simulink library "Code_Gen_lib"  (R2023a)
settings: Solver=VariableStepAuto  StartTime=0.0  StopTime=10.0  RelTol=1e-3
libraries: Autonomous_lib x1, Disabled_lib x1, Swerve_Drive_lib x1, Teleop_lib x1, Test_lib x1
settings Model: Creator=FIRSTMentor  LastModifiedBy=FIRSTMentor

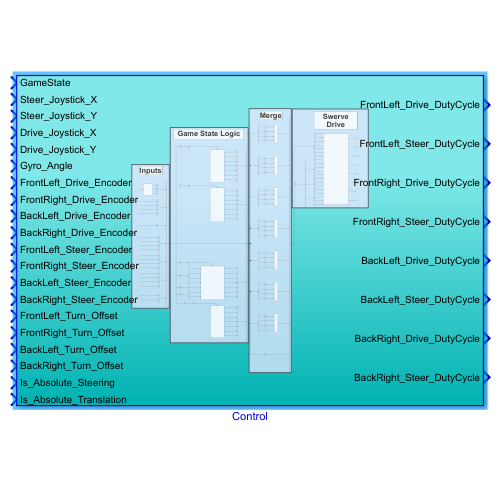
[thumbnail: Simulink's stored preview of the top-level diagram]
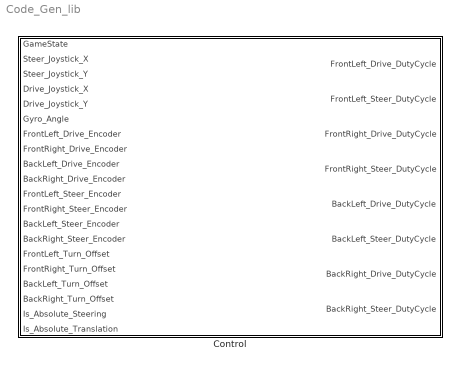
== system Code_Gen_lib ==
  Control : Subsystem

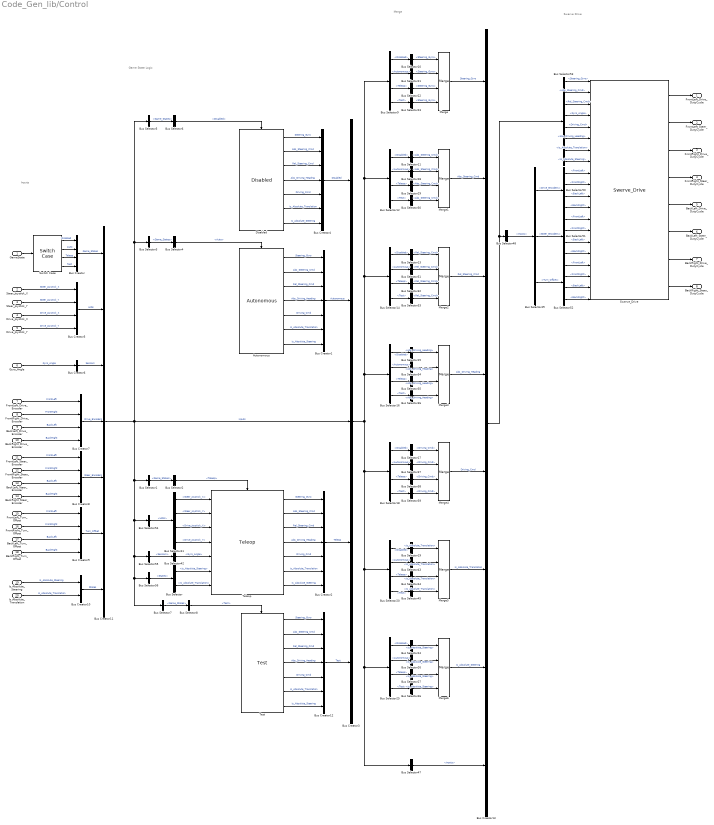
== system Code_Gen_lib/Control ==
  note: Game State Logic
  note: Merge
  note: Swerve Drive
  note: Inputs
  GameState : Inport
  Steer_Joystick_X : Inport  Port=2
  Steer_Joystick_Y : Inport  Port=3
  Drive_Joystick_X : Inport  Port=4
  Drive_Joystick_Y : Inport  Port=5
  Gyro_Angle : Inport  Port=6
  FrontLeft_Drive_Encoder : Inport  Port=7
  FrontRight_Drive_Encoder : Inport  Port=8
  BackLeft_Drive_Encoder : Inport  Port=9
  BackRight_Drive_Encoder : Inport  Port=10
  FrontLeft_Steer_Encoder : Inport  Port=11
  FrontRight_Steer_Encoder : Inport  Port=12
  BackLeft_Steer_Encoder : Inport  Port=13
  BackRight_Steer_Encoder : Inport  Port=14
  FrontLeft_Turn_Offset : Inport  Port=15
  FrontRight_Turn_Offset : Inport  Port=16
  BackLeft_Turn_Offset : Inport  Port=17
  BackRight_Turn_Offset : Inport  Port=18
  Is_Absolute_Steering : Inport  Port=19
  Is_Absolute_Translation : Inport  Port=20
  Autonomous : Autonomous_lib/Autonomous  SystemSampleTime=-1  VariantActivationTime=update diagram  Latency=0  AutoFrameSizeCalculation=off
  Bus Creator{,5,7..9} (5 alike) : BusCreator  Inputs=4
  Bus Creator{1..2,4,11..12} (5 alike) : BusCreator  Inputs=7
  Bus Creator10 : BusCreator  Inputs=2
  Bus Creator13 : BusCreator  Inputs=8
  Bus Creator3 : BusCreator  Inputs=5
  Bus Creator6 : BusCreator  Inputs=1
  Bus Selector : BusSelector  OutputSignals=Is_Absolute_Steering,Is_Absolute_Translation
  Bus Selector{1,3,5,7} (4 alike) : BusSelector  OutputSignals=Game_States
  Bus Selector{10,21..23} (4 alike) : BusSelector  OutputSignals=Steering_Gyro
  Bus Selector{11,28..30} (4 alike) : BusSelector  OutputSignals=Abs_Steering_Cmd
  Bus Selector{9,12,14,16,18,20,25} (7 alike) : BusSelector  OutputSignals=Disabled,Autonomous,Teleop,Test
  Bus Selector{13,31..33} (4 alike) : BusSelector  OutputSignals=Rel_Steering_Cmd
  Bus Selector{15,34..36} (4 alike) : BusSelector  OutputSignals=Abs_Driving_Heading
  Bus Selector{17,37..39} (4 alike) : BusSelector  OutputSignals=Driving_Cmd
  Bus Selector{19,43..45} (4 alike) : BusSelector  OutputSignals=Is_Absolute_Translation
  Bus Selector2 : BusSelector  OutputSignals=Teleop
  Bus Selector{24,26..27,46} (4 alike) : BusSelector  OutputSignals=Is_Absolute_Steering
  Bus Selector4 : BusSelector  OutputSignals=Auto
  Bus Selector41 : BusSelector  OutputSignals=Steer_Joystick_X,Steer_Joystick_Y,Drive_Joystick_X,Drive_Joystick_Y
  Bus Selector42 : BusSelector  OutputSignals=Gyro_Angle
  Bus Selector47 : BusSelector  OutputSignals=Inputs
  Bus Selector48 : BusSelector  OutputSignals=Inputs
  Bus Selector49 : BusSelector  OutputSignals=Drive_Encoders,Steer_Encoders,Turn_Offset
  Bus Selector50 : BusSelector  OutputSignals=FrontLeft,FrontRight,BackLeft,BackRight
  Bus Selector51 : BusSelector  OutputSignals=FrontLeft,FrontRight,BackLeft,BackRight
  Bus Selector52 : BusSelector  OutputSignals=FrontLeft,FrontRight,BackLeft,BackRight
  Bus Selector53 : BusSelector  OutputSignals=Steering_Gyro,Abs_Steering_Cmd,Rel_Steering_Cmd,Inputs.Sensors.Gyro_Angle,Driving_Cmd,Abs_Driving_Heading,Is_Absolute_Translation,Is_Absolute_Steering
  Bus Selector54 : BusSelector  OutputSignals=HIDs
  Bus Selector55 : BusSelector  OutputSignals=Sensors
  Bus Selector56 : BusSelector  OutputSignals=States
  Bus Selector6 : BusSelector  OutputSignals=Disabled
  Bus Selector8 : BusSelector  OutputSignals=Test
  Disabled : Disabled_lib/Disabled  SystemSampleTime=-1  VariantActivationTime=update diagram  Latency=0  AutoFrameSizeCalculation=off
  Merge{,1..6} (7 alike) : Merge  Inputs=4
  Swerve_Drive : Swerve_Drive_lib/Swerve_Drive  SystemSampleTime=-1  VariantActivationTime=update diagram  Latency=0  AutoFrameSizeCalculation=off
  Switch Case : SwitchCase  CaseConditions={0,1,2}
  Teleop : Teleop_lib/Teleop  SystemSampleTime=-1  VariantActivationTime=update diagram  Latency=0  AutoFrameSizeCalculation=off
  Test : Test_lib/Test  SystemSampleTime=-1  VariantActivationTime=update diagram  Latency=0  AutoFrameSizeCalculation=off
  FrontLeft_Drive_DutyCycle : Outport
  FrontLeft_Steer_DutyCycle : Outport  Port=2
  FrontRight_Drive_DutyCycle : Outport  Port=3
  FrontRight_Steer_DutyCycle : Outport  Port=4
  BackLeft_Drive_DutyCycle : Outport  Port=5
  BackLeft_Steer_DutyCycle : Outport  Port=6
  BackRight_Drive_DutyCycle : Outport  Port=7
  BackRight_Steer_DutyCycle : Outport  Port=8
  wires:
  Teleop/1 -> Bus Creator2/1  "Steering_Gyro"
  Teleop/2 -> Bus Creator2/2  "Abs_Steering_Cmd"
  Teleop/3 -> Bus Creator2/3  "Rel_Steering_Cmd"
  Teleop/4 -> Bus Creator2/4  "Abs_Driving_Heading"
  Teleop/5 -> Bus Creator2/5  "Driving_Cmd"
  Bus Creator4/1 -> Bus Creator3/1  "Disabled"
  Bus Creator1/1 -> Bus Creator3/2  "Autonomous"
  Bus Creator2/1 -> Bus Creator3/4  "Teleop"
  Switch Case/1 -> Bus Creator/1  "Disabled"
  Switch Case/2 -> Bus Creator/2  "Auto"
  Switch Case/3 -> Bus Creator/3  "Teleop"
  GameState/1 -> Switch Case/1
  Bus Creator12/1 -> Bus Creator3/5  "Test"
  Switch Case/4 -> Bus Creator/4  "Test"
  Steer_Joystick_Y/1 -> Bus Creator5/2  "Steer_Joystick_Y"
  Steer_Joystick_X/1 -> Bus Creator5/1  "Steer_Joystick_X"
  Drive_Joystick_X/1 -> Bus Creator5/3  "Drive_Joystick_X"
  Drive_Joystick_Y/1 -> Bus Creator5/4  "Drive_Joystick_Y"
  Gyro_Angle/1 -> Bus Creator6/1  "Gyro_Angle"
  Bus Creator5/1 -> Bus Creator11/2  "HIDs"
  Bus Creator6/1 -> Bus Creator11/3  "Sensors"
  FrontLeft_Drive_Encoder/1 -> Bus Creator7/1  "FrontLeft"
  FrontRight_Drive_Encoder/1 -> Bus Creator7/2  "FrontRight"
  BackLeft_Drive_Encoder/1 -> Bus Creator7/3  "BackLeft"
  BackRight_Drive_Encoder/1 -> Bus Creator7/4  "BackRight"
  FrontLeft_Steer_Encoder/1 -> Bus Creator8/1  "FrontLeft"
  BackLeft_Steer_Encoder/1 -> Bus Creator8/3  "BackLeft"
  BackRight_Steer_Encoder/1 -> Bus Creator8/4  "BackRight"
  FrontRight_Steer_Encoder/1 -> Bus Creator8/2  "FrontRight"
  Bus Creator7/1 -> Bus Creator11/4  "Drive_Encoders"
  Bus Creator8/1 -> Bus Creator11/5  "Steer_Encoders"
  FrontLeft_Turn_Offset/1 -> Bus Creator9/1  "FrontLeft"
  FrontRight_Turn_Offset/1 -> Bus Creator9/2  "FrontRight"
  BackLeft_Turn_Offset/1 -> Bus Creator9/3  "BackLeft"
  BackRight_Turn_Offset/1 -> Bus Creator9/4  "BackRight"
  Bus Creator9/1 -> Bus Creator11/6  "Turn_Offset"
  Is_Absolute_Steering/1 -> Bus Creator10/1  "Is_Absolute_Steering"
  Is_Absolute_Translation/1 -> Bus Creator10/2  "Is_Absolute_Translation"
  Bus Creator10/1 -> Bus Creator11/7  "States"
  Bus Selector54/1 -> Bus Selector41/1  "<HIDs>"
  Bus Selector41/1 -> Teleop/1  "<Steer_Joystick_X>"
  Bus Selector41/2 -> Teleop/2  "<Steer_Joystick_Y>"
  Bus Selector41/3 -> Teleop/3  "<Drive_Joystick_X>"
  Bus Selector41/4 -> Teleop/4  "<Drive_Joystick_Y>"
  Bus Selector55/1 -> Bus Selector42/1  "<Sensors>"
  Bus Selector42/1 -> Teleop/5  "<Gyro_Angle>"
  Swerve_Drive/1 -> FrontLeft_Drive_DutyCycle/1
  Swerve_Drive/2 -> FrontLeft_Steer_DutyCycle/1
  Swerve_Drive/3 -> FrontRight_Drive_DutyCycle/1
  Swerve_Drive/4 -> FrontRight_Steer_DutyCycle/1
  Swerve_Drive/5 -> BackLeft_Drive_DutyCycle/1
  Swerve_Drive/6 -> BackLeft_Steer_DutyCycle/1
  Swerve_Drive/8 -> BackRight_Steer_DutyCycle/1
  Swerve_Drive/7 -> BackRight_Drive_DutyCycle/1
  Teleop/6 -> Bus Creator2/6  "Is_Absolute_Translation"
  Teleop/7 -> Bus Creator2/7  "Is_Absolute_Steering"
  Bus Selector56/1 -> Bus Selector/1  "<States>"
  Bus Selector/1 -> Teleop/6  "<Is_Absolute_Steering>"
  Bus Selector/2 -> Teleop/7  "<Is_Absolute_Translation>"
  Autonomous/2 -> Bus Creator1/2  "Abs_Steering_Cmd"
  Autonomous/4 -> Bus Creator1/4  "Abs_Driving_Heading"
  Autonomous/1 -> Bus Creator1/1  "Steering_Gyro"
  Autonomous/5 -> Bus Creator1/5  "Driving_Cmd"
  Autonomous/7 -> Bus Creator1/7  "Is_Absolute_Steering"
  Autonomous/3 -> Bus Creator1/3  "Rel_Steering_Cmd"
  Autonomous/6 -> Bus Creator1/6  "Is_Absolute_Translation"
  Disabled/2 -> Bus Creator4/2  "Abs_Steering_Cmd"
  Disabled/4 -> Bus Creator4/4  "Abs_Driving_Heading"
  Disabled/1 -> Bus Creator4/1  "Steering_Gyro"
  Disabled/5 -> Bus Creator4/5  "Driving_Cmd"
  Disabled/7 -> Bus Creator4/7  "Is_Absolute_Steering"
  Disabled/3 -> Bus Creator4/3  "Rel_Steering_Cmd"
  Disabled/6 -> Bus Creator4/6  "Is_Absolute_Translation"
  Test/2 -> Bus Creator12/2  "Abs_Steering_Cmd"
  Test/4 -> Bus Creator12/4  "Abs_Driving_Heading"
  Test/1 -> Bus Creator12/1  "Steering_Gyro"
  Test/5 -> Bus Creator12/5  "Driving_Cmd"
  Test/7 -> Bus Creator12/7  "Is_Absolute_Steering"
  Test/3 -> Bus Creator12/3  "Rel_Steering_Cmd"
  Test/6 -> Bus Creator12/6  "Is_Absolute_Translation"
  Bus Creator/1 -> Bus Creator11/1  "Game_States"
  Bus Selector1/1 -> Bus Selector2/1  "<Game_States>"
  Bus Selector2/1 -> Teleop/Action  "<Teleop>"
  Bus Selector3/1 -> Bus Selector4/1  "<Game_States>"
  Bus Selector4/1 -> Autonomous/Action  "<Auto>"
  Bus Selector5/1 -> Bus Selector6/1  "<Game_States>"
  Bus Selector6/1 -> Disabled/Action  "<Disabled>"
  Bus Selector7/1 -> Bus Selector8/1  "<Game_States>"
  Bus Selector8/1 -> Test/Action  "<Test>"
  Bus Creator11/1 -> Bus Selector1/1, Bus Selector54/1, Bus Selector55/1, Bus Selector56/1, Bus Selector7/1, Bus Selector5/1, Bus Selector3/1, Bus Creator3/3  "Inputs"
  Bus Selector9/1 -> Bus Selector10/1  "<Disabled>"
  Bus Selector10/1 -> Merge/1  "<Steering_Gyro>"
  Bus Selector11/1 -> Merge1/1  "<Abs_Steering_Cmd>"
  Bus Selector12/1 -> Bus Selector11/1  "<Disabled>"
  Bus Selector13/1 -> Merge2/1  "<Rel_Steering_Cmd>"
  Bus Selector14/1 -> Bus Selector13/1  "<Disabled>"
  Bus Selector15/1 -> Merge3/1  "<Abs_Driving_Heading>"
  Bus Selector16/1 -> Bus Selector15/1  "<Disabled>"
  Bus Selector17/1 -> Merge4/1  "<Driving_Cmd>"
  Bus Selector18/1 -> Bus Selector17/1  "<Disabled>"
  Bus Selector19/1 -> Merge5/1  "<Is_Absolute_Translation>"
  Bus Selector20/1 -> Bus Selector19/1  "<Disabled>"
  Bus Selector21/1 -> Merge/2  "<Steering_Gyro>"
  Bus Selector9/2 -> Bus Selector21/1  "<Autonomous>"
  Bus Selector22/1 -> Merge/3  "<Steering_Gyro>"
  Bus Selector9/3 -> Bus Selector22/1  "<Teleop>"
  Bus Selector23/1 -> Merge/4  "<Steering_Gyro>"
  Bus Selector9/4 -> Bus Selector23/1  "<Test>"
  Bus Selector25/1 -> Bus Selector24/1  "<Disabled>"
  Bus Selector24/1 -> Merge6/1  "<Is_Absolute_Steering>"
  Bus Creator3/1 -> Bus Selector16/1, Bus Selector14/1, Bus Selector12/1, Bus Selector9/1, Bus Selector47/1, Bus Selector25/1, Bus Selector20/1, Bus Selector18/1
  Bus Selector12/2 -> Bus Selector28/1  "<Autonomous>"
  Bus Selector28/1 -> Merge1/2  "<Abs_Steering_Cmd>"
  Bus Selector12/3 -> Bus Selector29/1  "<Teleop>"
  Bus Selector29/1 -> Merge1/3  "<Abs_Steering_Cmd>"
  Bus Selector12/4 -> Bus Selector30/1  "<Test>"
  Bus Selector30/1 -> Merge1/4  "<Abs_Steering_Cmd>"
  Bus Selector31/1 -> Merge2/2  "<Rel_Steering_Cmd>"
  Bus Selector14/2 -> Bus Selector31/1  "<Autonomous>"
  Bus Selector32/1 -> Merge2/3  "<Rel_Steering_Cmd>"
  Bus Selector14/3 -> Bus Selector32/1  "<Teleop>"
  Bus Selector33/1 -> Merge2/4  "<Rel_Steering_Cmd>"
  Bus Selector14/4 -> Bus Selector33/1  "<Test>"
  Bus Selector16/2 -> Bus Selector34/1  "<Autonomous>"
  Bus Selector34/1 -> Merge3/2  "<Abs_Driving_Heading>"
  Bus Selector16/3 -> Bus Selector35/1  "<Teleop>"
  Bus Selector35/1 -> Merge3/3  "<Abs_Driving_Heading>"
  Bus Selector16/4 -> Bus Selector36/1  "<Test>"
  Bus Selector36/1 -> Merge3/4  "<Abs_Driving_Heading>"
  Bus Selector18/2 -> Bus Selector37/1  "<Autonomous>"
  Bus Selector37/1 -> Merge4/2  "<Driving_Cmd>"
  Bus Selector18/3 -> Bus Selector38/1  "<Teleop>"
  Bus Selector38/1 -> Merge4/3  "<Driving_Cmd>"
  Bus Selector18/4 -> Bus Selector39/1  "<Test>"
  Bus Selector39/1 -> Merge4/4  "<Driving_Cmd>"
  Bus Selector20/2 -> Bus Selector43/1  "<Autonomous>"
  Bus Selector43/1 -> Merge5/2  "<Is_Absolute_Translation>"
  Bus Selector45/1 -> Merge5/4  "<Is_Absolute_Translation>"
  Bus Selector20/4 -> Bus Selector45/1  "<Test>"
  Bus Selector20/3 -> Bus Selector44/1  "<Teleop>"
  Bus Selector44/1 -> Merge5/3  "<Is_Absolute_Translation>"
  Bus Selector25/2 -> Bus Selector26/1  "<Autonomous>"
  Bus Selector26/1 -> Merge6/2  "<Is_Absolute_Steering>"
  Bus Selector25/4 -> Bus Selector46/1  "<Test>"
  Bus Selector25/3 -> Bus Selector27/1  "<Teleop>"
  Bus Selector46/1 -> Merge6/4  "<Is_Absolute_Steering>"
  Bus Selector27/1 -> Merge6/3  "<Is_Absolute_Steering>"
  Merge/1 -> Bus Creator13/1  "Steering_Gyro"
  Merge1/1 -> Bus Creator13/2  "Abs_Steering_Cmd"
  Merge2/1 -> Bus Creator13/3  "Rel_Steering_Cmd"
  Merge3/1 -> Bus Creator13/4  "Abs_Driving_Heading"
  Merge4/1 -> Bus Creator13/5  "Driving_Cmd"
  Merge5/1 -> Bus Creator13/6  "Is_Absolute_Translation"
  Merge6/1 -> Bus Creator13/7  "Is_Absolute_Steering"
  Bus Selector47/1 -> Bus Creator13/8  "<Inputs>"
  Bus Creator13/1 -> Bus Selector48/1, Bus Selector53/1
  Bus Selector48/1 -> Bus Selector49/1  "<Inputs>"
  Bus Selector49/1 -> Bus Selector50/1  "<Drive_Encoders>"
  Bus Selector49/2 -> Bus Selector51/1  "<Steer_Encoders>"
  Bus Selector49/3 -> Bus Selector52/1  "<Turn_Offset>"
  Bus Selector53/1 -> Swerve_Drive/1  "<Steering_Gyro>"
  Bus Selector53/2 -> Swerve_Drive/2  "<Abs_Steering_Cmd>"
  Bus Selector53/3 -> Swerve_Drive/3  "<Rel_Steering_Cmd>"
  Bus Selector53/5 -> Swerve_Drive/5  "<Driving_Cmd>"
  Bus Selector53/7 -> Swerve_Drive/7  "<Is_Absolute_Translation>"
  Bus Selector53/8 -> Swerve_Drive/8  "<Is_Absolute_Steering>"
  Bus Selector52/4 -> Swerve_Drive/20  "<BackRight>"
  Bus Selector52/3 -> Swerve_Drive/19  "<BackLeft>"
  Bus Selector52/2 -> Swerve_Drive/18  "<FrontRight>"
  Bus Selector52/1 -> Swerve_Drive/17  "<FrontLeft>"
  Bus Selector51/4 -> Swerve_Drive/16  "<BackRight>"
  Bus Selector51/3 -> Swerve_Drive/15  "<BackLeft>"
  Bus Selector51/2 -> Swerve_Drive/14  "<FrontRight>"
  Bus Selector51/1 -> Swerve_Drive/13  "<FrontLeft>"
  Bus Selector50/4 -> Swerve_Drive/12  "<BackRight>"
  Bus Selector50/3 -> Swerve_Drive/11  "<BackLeft>"
  Bus Selector50/2 -> Swerve_Drive/10  "<FrontRight>"
  Bus Selector50/1 -> Swerve_Drive/9  "<FrontLeft>"
  Bus Selector53/4 -> Swerve_Drive/4  "<Gyro_Angle>"
  Bus Selector53/6 -> Swerve_Drive/6  "<Abs_Driving_Heading>"
